simulink model "GesamtsystemAltV3_IRS"  (R2018b)
settings: Solver=FixedStepDiscrete  StartTime=0.0  StopTime=1  RelTol=1e-3  EnableMultiTasking=on
libraries: commutil2 x12, c2833xlib x10, c280xlib x8, powerlib_extras x2, c2000lib x1, dspstat3 x1
(part 3 of 3)

== matlab function GesamtsystemAltV3_IRS/Subsystem/getAngle2/Messung des absoluten Winkels - Auswertung der Encodersignale/MATLAB Function2 ==
  data: u1 input; u1alt input; u2 input; u2alt input; y output; yalt input double; RL output
function [y, RL] = fcn(u1, u1alt, u2, u2alt, yalt)

y = 1;
RL = 1;

if u1alt == 0 && u2alt == 0 && u1 == 0 && u2 == 0
    y = yalt;
end

if u1alt == 0 && u2alt == 0 && u1 == 0 && u2 == 1
    y = 1;
end

if u1alt == 0 && u2alt == 0 && u1 == 1 && u2 == 0
    y = -1;
end

% if u1alt == 0 && u2alt == 0 && u1 == 1 && u2 == 1
%     y = yalt;   % nicht möglich
% end

if u1alt == 0 && u2alt == 1 && u1 == 0 && u2 == 0
    y = -1;
end

if u1alt == 0 && u2alt == 1 && u1 == 0 && u2 == 1
    y = yalt;
end

% if u1alt == 0 && u2alt == 1 && u1 == 1 && u2 == 0
%     y = yalt;   % nicht möglich
% end

if u1alt == 0 && u2alt == 1 && u1 == 1 && u2 == 1
    y = 1;
end

if u1alt == 1 && u2alt == 0 && u1 == 0 && u2 == 0
    y = 1;
end

% if u1alt == 1 && u2alt == 0 && u1 == 0 && u2 == 1
%     y = yalt;   % nicht möglich
% end

if u1alt == 1 && u2alt == 0 && u1 == 1 && u2 == 0
    y = yalt;
end

if u1alt == 1 && u2alt == 0 && u1 == 1 && u2 == 1
    y = -1;
end

% if u1alt == 1 && u2alt == 1 && u1 == 0 && u2 == 0
%     y = yalt;   % nicht möglich
% end

if u1alt == 1 && u2alt == 1 && u1 == 0 && u2 == 1
    y = -1;
end

if u1alt == 1 && u2alt == 1 && u1 == 1 && u2 == 0
    y = 1;
end

if u1alt == 1 && u2alt == 1 && u1 == 1 && u2 == 1
    y = yalt;
end

if y == 1
    RL = 1;
else
    RL = 0;
end

== matlab function GesamtsystemAltV3_IRS/Subsystem/getAngle2/Messung des absoluten Winkels - Auswertung der Encodersignale/MATLAB Function3 ==
  data: u input; y output; yalt input
function y = fcn(u, yalt)

y = yalt + u;
